simulink model "simulate_lqr"  (R2020a)
settings: Solver=VariableStepAuto  StartTime=0.0  StopTime=4  RelTol=1e-3
values from neighbouring files (symbols this model uses):
  A = [0, 1; g/L, 0]    [main.m]    (also in plant.m = [0, 1; -g/L, 0])
  B = [0; 1/(m * L^2)]    [main.m]    (also in plant.m = [0; 1/m])
  C = [1, 0]    [main.m]    (also in plant.m)
undefined symbols (not defined in the file or in its folder): K
settings Model: Creator=Takumi  LastModifiedBy=Takumi

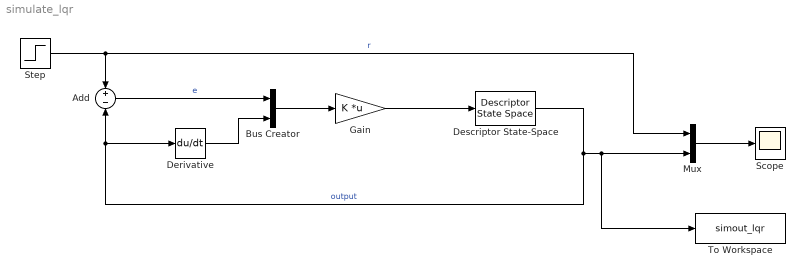
== system simulate_lqr ==
  Add : Sum  Inputs=+-
  Bus Creator : BusCreator  Inputs=2
  Derivative : Derivative
  Descriptor State-Space : DescriptorStateSpace  E=eye(2)  A=A  B=B  C=C  D=0  InitialCondition=0  ContinuousStateAttributes='state'
  Gain : Gain  Gain=K  Multiplication=Matrix(K*u)
  Mux : Mux  Inputs=2
  Scope : Scope
  Step : Step  SampleTime=0
  To Workspace : ToWorkspace  VariableName=simout_lqr  SaveFormat=Timeseries  SampleTime=-1
  wires:
  Descriptor State-Space/1 -> To Workspace/1, Mux/2, Derivative/1, Add/2  "output"
  Step/1 -> Add/1, Mux/1  "r"
  Add/1 -> Bus Creator/1  "e"
  Mux/1 -> Scope/1
  Gain/1 -> Descriptor State-Space/1
  Derivative/1 -> Bus Creator/2
  Bus Creator/1 -> Gain/1
